simulink model "fuzzycontrol"  (Simulink 5.0)
settings: Solver=ode45  StartTime=0.0  StopTime=100  RelTol=1e-3
PreLoadFcn:
  | new=readfis('new.fis');
InitFcn:
  | init_c
values from neighbouring files (symbols this model uses):
  a = 0.0125463709677    [lastfuzzy.mat]
  dzcv = 0.0079311    [lastfuzzy.mat]
  fc = 0.9    [lastfuzzy.mat]
  fp = 0.000107443    [lastfuzzy.mat]
  fs = 2.28133    [lastfuzzy.mat]
  g = 9.81    [lastfuzzy.mat]
  j = 0.0135735    [lastfuzzy.mat]
  l = 0.04    [lastfuzzy.mat]
  mi = 0.0496    [lastfuzzy.mat]
  xc = 2.5    [lastfuzzy.mat]
  yc = 2.5    [lastfuzzy.mat]
libraries: fuzblock x2
settings Model: LastModifiedBy=AD  BooleanDataType=off

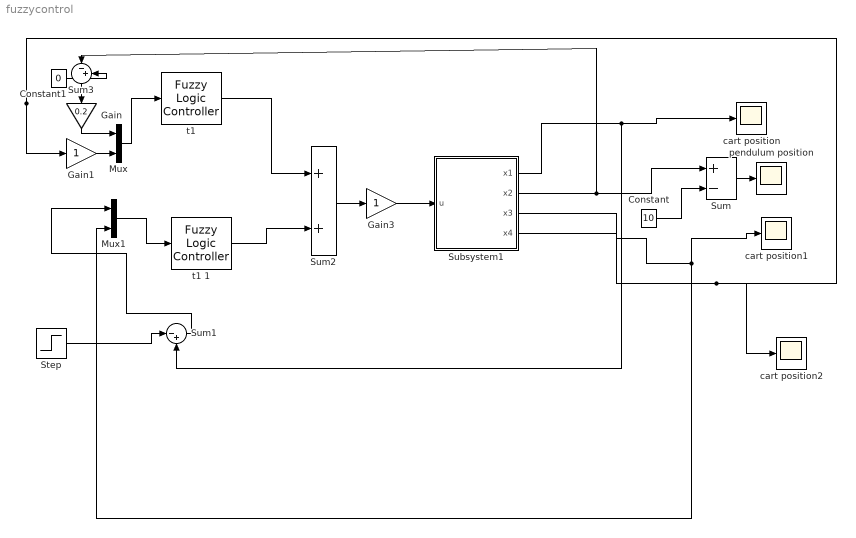
== system fuzzycontrol ==
  Constant : Constant  Value=10
  Constant1 : Constant  Value=0
  Gain : Gain  Orientation=down  Gain=0.2  SaturateOnIntegerOverflow=on
  Gain1 : Gain  SaturateOnIntegerOverflow=on
  Gain3 : Gain  SaturateOnIntegerOverflow=on
  Mux : Mux  Inputs=2
  Mux1 : Mux  Inputs=2
  Step : Step  SampleTime=0
  Subsystem1 : Subsystem
  Sum : Sum  Inputs=|+-  SaturateOnIntegerOverflow=on
  Sum1 : Sum  Inputs=|-+  SaturateOnIntegerOverflow=on
  Sum2 : Sum  SaturateOnIntegerOverflow=on
  Sum3 : Sum  Orientation=down  Inputs=|-+  SaturateOnIntegerOverflow=on
  cart position : Scope
      settings: TimeRange=100  YMin=0.826  YMax=0.843
  cart position1 : Scope
      settings: TimeRange=100  YMin=0.0045  YMax=0.013
  cart position2 : Scope
      settings: YMin=-7  YMax=7  SaveName=ScopeData3
  pendulum position : Scope
      settings: YMin=-9  YMax=-4.75  SaveName=ScopeData4
  "t1 " : fuzblock/Fuzzy Logic  Controller  fis=new
  t1 1 : fuzblock/Fuzzy Logic  Controller  fis=new
  wires:
  Sum/1 -> pendulum position/1
  Constant/1 -> Sum/2
  Subsystem1/3(x3) -> cart position1/1, Mux1/2
  Subsystem1/4(x4) -> cart position2/1, Gain1/1
  Subsystem1/1(x1) -> cart position/1, Sum1/2
  Subsystem1/2(x2) -> Sum/1, Sum3/1
  Mux1/1 -> t1 1/1
  Sum1/1 -> Mux1/1
  Mux/1 -> "t1 "/1
  Step/1 -> Sum1/1
  Constant1/1 -> Sum3/2
  Sum3/1 -> Gain/1
  Sum2/1 -> Gain3/1
  "t1 "/1 -> Sum2/1
  Gain3/1 -> Subsystem1/1(u)
  Gain1/1 -> Mux/2
  Gain/1 -> Mux/1
  t1 1/1 -> Sum2/2

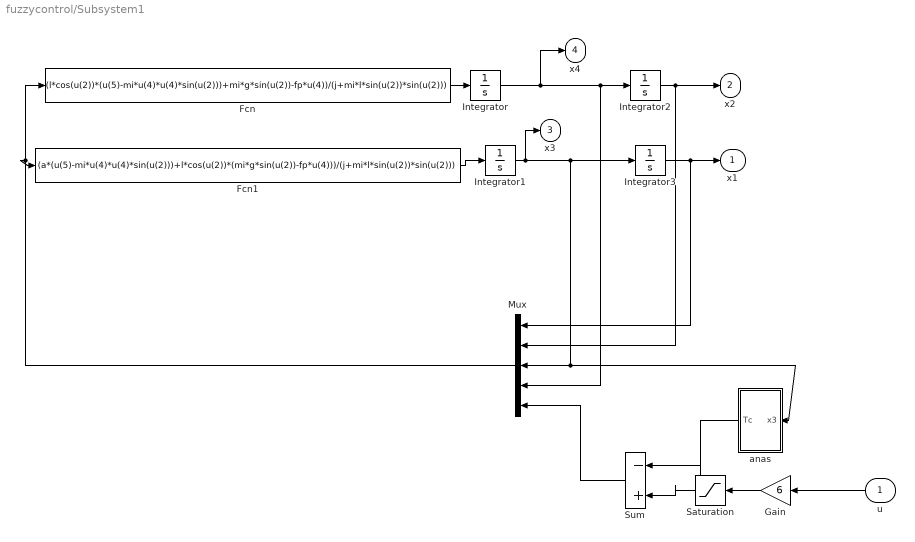
== system fuzzycontrol/Subsystem1 ==
  u : Inport  Orientation=left
  Fcn : Fcn  Expr=(l*cos(u(2))*(u(5)-mi*u(4)*u(4)*sin(u(2)))+mi*g*sin(u(2))-fp*u(4))/(j+mi*l*sin(u(2))*sin(u(2)))
  Fcn1 : Fcn  Expr=(a*(u(5)-mi*u(4)*u(4)*sin(u(2)))+l*cos(u(2))*(mi*g*sin(u(2))-fp*u(4)))/(j+mi*l*sin(u(2))*sin(u(2)))
  Gain : Gain  Orientation=left  Gain=6  SaturateOnIntegerOverflow=on
  Integrator{,1..3} (4 alike) : Integrator
  Mux : Mux  Orientation=left  Inputs=5
  Saturation : Saturate  Orientation=left  UpperLimit=17  LowerLimit=-17
  Sum : Sum  Orientation=left  Inputs=|-+  SaturateOnIntegerOverflow=on
  anas : Subsystem  Orientation=left
  x1 : Outport
  x2 : Outport  Port=2
  x3 : Outport  Port=3
  x4 : Outport  Port=4
  wires:
  Fcn/1 -> Integrator/1
  Fcn1/1 -> Integrator1/1
  Integrator/1 -> Integrator2/1, Mux/4, x4/1
  Integrator1/1 -> Integrator3/1, Mux/3, anas/1(x3), x3/1
  Integrator2/1 -> x2/1, Mux/2
  Integrator3/1 -> x1/1, Mux/1
  Mux/1 -> Fcn1/1, Fcn/1
  Sum/1 -> Mux/5
  Gain/1 -> Saturation/1
  Saturation/1 -> Sum/2
  u/1 -> Gain/1
  anas/1(Tc) -> Sum/1

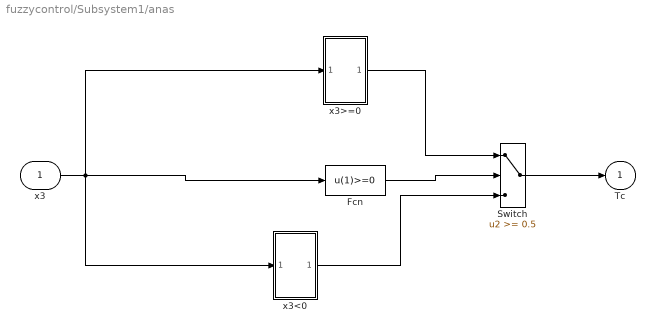
== system fuzzycontrol/Subsystem1/anas ==
  x3 : Inport
  Fcn : Fcn  Expr=u(1)>=0
  Switch : Switch  Threshold=0.5  SaturateOnIntegerOverflow=on
  x3<0 : Subsystem
  x3>=0 : Subsystem
  Tc : Outport
  wires:
  Switch/1 -> Tc/1
  Fcn/1 -> Switch/2
  x3/1 -> Fcn/1, x3>=0/1(In1), x3<0/1(In1)
  x3>=0/1(out1) -> Switch/1
  x3<0/1(out1) -> Switch/3

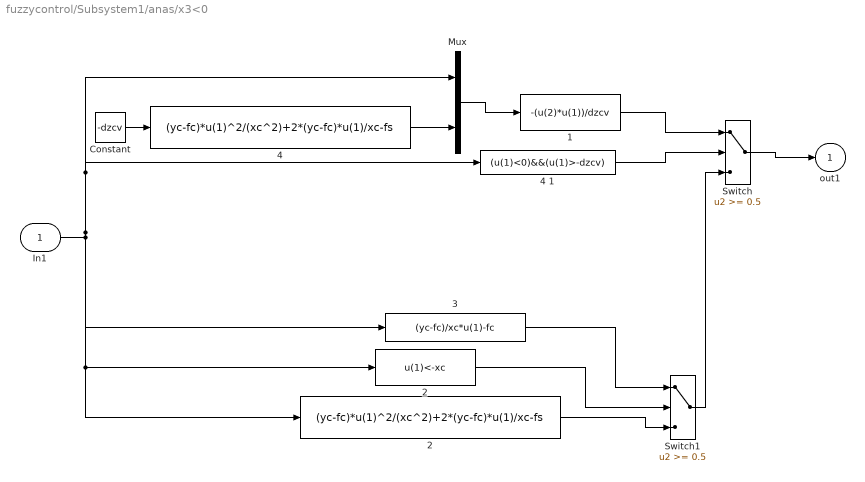
== system fuzzycontrol/Subsystem1/anas/x3<0 ==
  In1 : Inport
  1 : Fcn  Expr=-(u(2)*u(1))/dzcv
  2 : Fcn  Expr=u(1)<-xc
  "2 " : Fcn  Expr=(yc-fc)*u(1)^2/(xc^2)+2*(yc-fc)*u(1)/xc-fs
  3 : Fcn  Expr=(yc-fc)/xc*u(1)-fc
  "4 " : Fcn  Expr=(yc-fc)*u(1)^2/(xc^2)+2*(yc-fc)*u(1)/xc-fs
  4 1 : Fcn  Expr=(u(1)<0)&&(u(1)>-dzcv)
  Constant : Constant  Value=-dzcv
  Mux : Mux  Inputs=2
  Switch : Switch  Threshold=0.5  SaturateOnIntegerOverflow=on
  Switch1 : Switch  Threshold=0.5  SaturateOnIntegerOverflow=on
  out1 : Outport
  wires:
  1/1 -> Switch/1
  3/1 -> Switch1/1
  2/1 -> Switch1/2
  "2 "/1 -> Switch1/3
  Switch1/1 -> Switch/3
  Mux/1 -> 1/1
  "4 "/1 -> Mux/2
  In1/1 -> 3/1, 2/1, "2 "/1, Mux/1, 4 1/1
  Constant/1 -> "4 "/1
  4 1/1 -> Switch/2
  Switch/1 -> out1/1

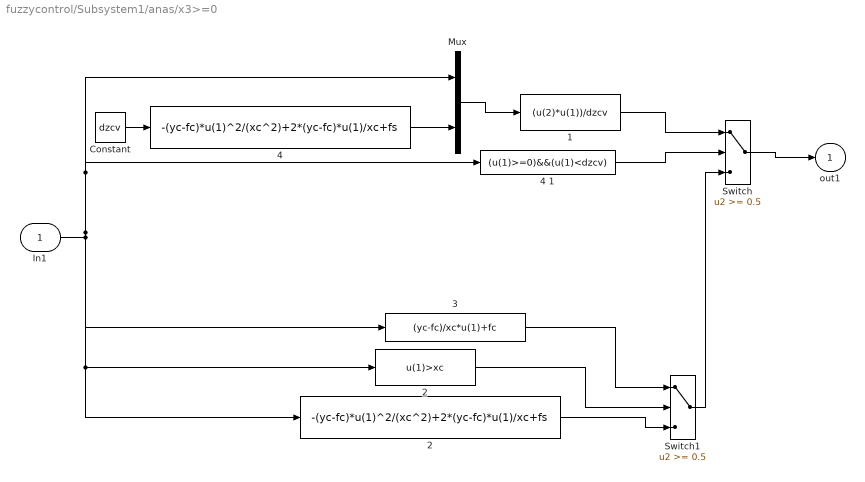
== system fuzzycontrol/Subsystem1/anas/x3>=0 ==
  In1 : Inport
  1 : Fcn  Expr=(u(2)*u(1))/dzcv
  2 : Fcn  Expr=u(1)>xc
  "2 " : Fcn  Expr=-(yc-fc)*u(1)^2/(xc^2)+2*(yc-fc)*u(1)/xc+fs
  3 : Fcn  Expr=(yc-fc)/xc*u(1)+fc
  "4 " : Fcn  Expr=-(yc-fc)*u(1)^2/(xc^2)+2*(yc-fc)*u(1)/xc+fs
  4 1 : Fcn  Expr=(u(1)>=0)&&(u(1)<dzcv)
  Constant : Constant  Value=dzcv
  Mux : Mux  Inputs=2
  Switch : Switch  Threshold=0.5  SaturateOnIntegerOverflow=on
  Switch1 : Switch  Threshold=0.5  SaturateOnIntegerOverflow=on
  out1 : Outport
  wires:
  1/1 -> Switch/1
  3/1 -> Switch1/1
  2/1 -> Switch1/2
  "2 "/1 -> Switch1/3
  Switch1/1 -> Switch/3
  Mux/1 -> 1/1
  "4 "/1 -> Mux/2
  In1/1 -> 3/1, 2/1, "2 "/1, Mux/1, 4 1/1
  Constant/1 -> "4 "/1
  4 1/1 -> Switch/2
  Switch/1 -> out1/1
